simulink model "FM"  (R2013a)
settings: Solver=ode45  StartTime=0.0  StopTime=12  FixedStep=1e-5  MaxStep=0.01  MinStep=0.01  RelTol=1e-3
values from neighbouring files (symbols this model uses):
  C = xlsread('Data.xlsx','C2:C101')    [Analysis.m]    (also in Quiz_3.m = 1e-06)
libraries: dspsigattribs x6, dspvision x6, dspestimation x1
settings Model: Creator=Mytea  LastModifiedBy=Mytea
settings SolverCC: InitialStep=0

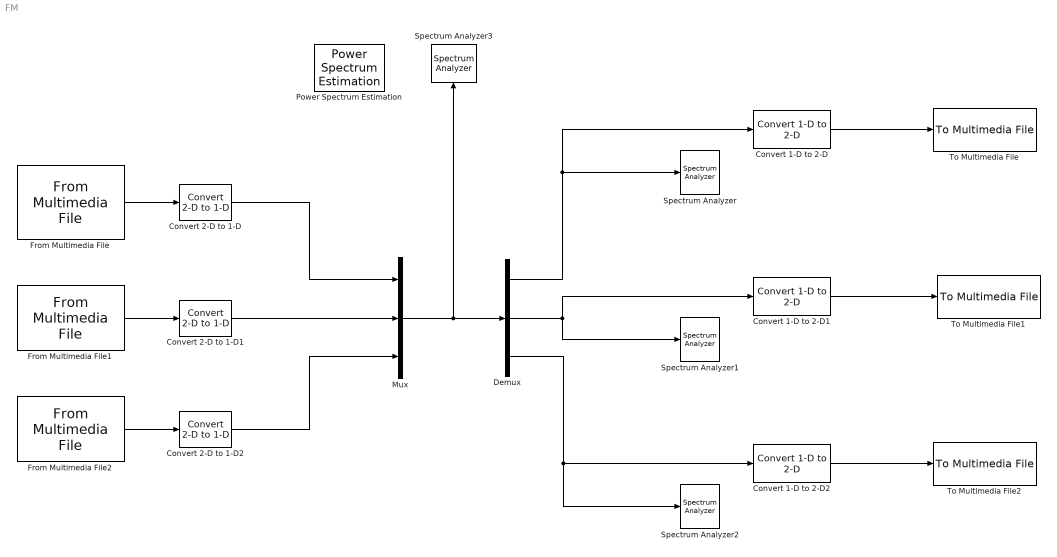
== system FM ==
  Convert 1-D to 2-D : dspsigattribs/Convert 1-D to 2-D  M=1024  N=2  frameBasedOut=off
  Convert 1-D to 2-D1 : dspsigattribs/Convert 1-D to 2-D  M=1024  N=2  frameBasedOut=off
  Convert 1-D to 2-D2 : dspsigattribs/Convert 1-D to 2-D  M=1024  N=2  frameBasedOut=off
  Convert 2-D to 1-D : dspsigattribs/Convert 2-D to 1-D
  Convert 2-D to 1-D1 : dspsigattribs/Convert 2-D to 1-D
  Convert 2-D to 1-D2 : dspsigattribs/Convert 2-D to 1-D
  Demux : Demux  Outputs=3
  From Multimedia File : dspvision/From Multimedia File  inputFilename=C:\Users\Mytea\Documents\MATLAB\mat995.wav  loop=on  numPlays=5  outputStreams=Audio only  videoDataType=single  audioDataType=double  inheritSampleTime=on  userDefinedSampleTime=1/30  noAudioOutput=off  isIntensityVideo=off  fourcc=RGB  colorVideoFormat=Separate color signals  outputEOF=off  dataOrg=Column-major  audioFrameSize=1024  computeAudioFrameSize=off  outSamplingMode=Sample based
  From Multimedia File1 : dspvision/From Multimedia File  inputFilename=C:\Users\Mytea\Documents\MATLAB\mat1011.wav  loop=on  numPlays=5  outputStreams=Audio only  videoDataType=single  audioDataType=double  inheritSampleTime=on  userDefinedSampleTime=1/30  noAudioOutput=off  isIntensityVideo=off  fourcc=RGB  colorVideoFormat=Separate color signals  outputEOF=off  dataOrg=Column-major  audioFrameSize=1024  computeAudioFrameSize=off  outSamplingMode=Sample based
  From Multimedia File2 : dspvision/From Multimedia File  inputFilename=C:\Users\Mytea\Documents\MATLAB\mat1015.wav  loop=on  numPlays=5  outputStreams=Audio only  videoDataType=single  audioDataType=double  inheritSampleTime=on  userDefinedSampleTime=1/30  noAudioOutput=off  isIntensityVideo=off  fourcc=RGB  colorVideoFormat=Separate color signals  outputEOF=off  dataOrg=Column-major  audioFrameSize=1024  computeAudioFrameSize=off  outSamplingMode=Sample based
  Mux : Mux  Inputs=3
  Power Spectrum Estimation : dspestimation/Power Spectrum Estimation
  Spectrum Analyzer{,1..3} (4 alike) : SpectrumAnalyzer
      settings: CopyFcn=scopeextensions.ScopeBlock.callback(gcbh, 'onBlockCopy', gcbh);  DeleteFcn=scopeextensions.ScopeBlock.callback(gcbh, 'onBlockDelete');  PreSaveFcn=scopeextensions.ScopeBlock.callback(gcbh, 'onModelSave');  NameChangeFcn=scopeextensions.ScopeBlock.callback(gcbh, 'onBlockRename');  CloseFcn=scopeextensions.ScopeBlock.callback(gcbh, 'onBlockClose');  PreDeleteFcn=scopeextensions.ScopeBlock.callback(gcbh, 'onBlockPreDelete');
  To Multimedia File : dspvision/To Multimedia File  outputFilename=C:\Users\Mytea\Documents\MATLAB\output1.wav  streamSelection=Audio only  videoCompressor=None (uncompressed)  audioCompressor=None (uncompressed)  imagePorts=Separate color signals  fileType=WAV  audioDatatype=16-bit integer  fourcc=RGB
  To Multimedia File1 : dspvision/To Multimedia File  outputFilename=C:\Users\Mytea\Documents\MATLAB\output2.wav  streamSelection=Audio only  videoCompressor=None (uncompressed)  audioCompressor=None (uncompressed)  imagePorts=Separate color signals  fileType=WAV  audioDatatype=16-bit integer  fourcc=RGB
  To Multimedia File2 : dspvision/To Multimedia File  outputFilename=C:\Users\Mytea\Documents\MATLAB\output3.wav  streamSelection=Audio only  videoCompressor=None (uncompressed)  audioCompressor=None (uncompressed)  imagePorts=Separate color signals  fileType=WAV  audioDatatype=16-bit integer  fourcc=RGB
  wires:
  Mux/1 -> Spectrum Analyzer3/1, Demux/1
  From Multimedia File/1 -> Convert 2-D to 1-D/1
  From Multimedia File1/1 -> Convert 2-D to 1-D1/1
  From Multimedia File2/1 -> Convert 2-D to 1-D2/1
  Demux/1 -> Convert 1-D to 2-D/1, Spectrum Analyzer/1
  Demux/2 -> Spectrum Analyzer1/1, Convert 1-D to 2-D1/1
  Convert 2-D to 1-D1/1 -> Mux/2
  Convert 2-D to 1-D2/1 -> Mux/3
  Convert 2-D to 1-D/1 -> Mux/1
  Convert 1-D to 2-D/1 -> To Multimedia File/1
  Convert 1-D to 2-D1/1 -> To Multimedia File1/1
  Convert 1-D to 2-D2/1 -> To Multimedia File2/1
  Demux/3 -> Spectrum Analyzer2/1, Convert 1-D to 2-D2/1
